simulink model "problem3"  (R2020b)
settings: Solver=VariableStepAuto  StartTime=0.0  StopTime=10.0  RelTol=1e-3
settings Model: Creator=Hp  LastModifiedBy=Makrand Raut Dessai

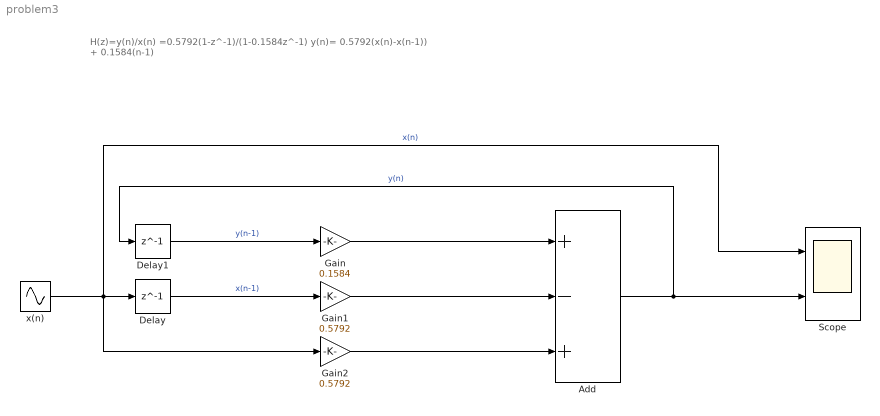
== system problem3 ==
  note: H(z)=y(n)/x(n) =0.5792(1-z^-1)/(1-0.1584z^-1)
      | y(n)= 0.5792(x(n)-x(n-1)) + 0.1584(n-1)
  Add : Sum  Inputs=+-+
  Delay : Delay  DelayLength=1
  Delay1 : Delay  DelayLength=1
  Gain : Gain  Gain=0.1584
  Gain1 : Gain  Gain=0.5792
  Gain2 : Gain  Gain=0.5792
  Scope : Scope  NumInputPorts=2
  x(n) : Sin  SampleTime=0
  wires:
  Add/1 -> Delay1/1, Scope/2  "y(n)"
  Delay1/1 -> Gain/1  "y(n-1)"
  Gain/1 -> Add/1
  Delay/1 -> Gain1/1  "x(n-1)"
  Gain1/1 -> Add/2
  Gain2/1 -> Add/3
  x(n)/1 -> Scope/1, Gain2/1, Delay/1  "x(n)"
